simulink model "H_Bridge"  (R2022a)
settings: Solver=VariableStepAuto  StartTime=0.0  StopTime=.06  RelTol=1e-3
libraries: spsVoltageMeasurementLib x2, spsSeriesRLCBranchLib x1, slpidlib x1, spsPVArrayLib x1, spsCurrentMeasurementLib x1, spspowerguiLib x1
settings Model: Creator=micha  LastModifiedBy=micha
settings DataIOCC: ReturnWorkspaceOutputs=off

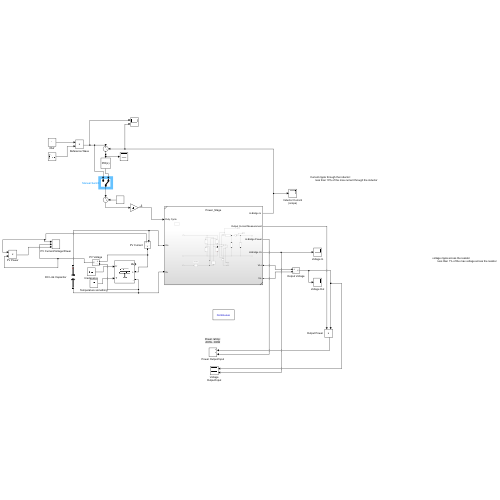
[thumbnail: Simulink's stored preview of the top-level diagram]
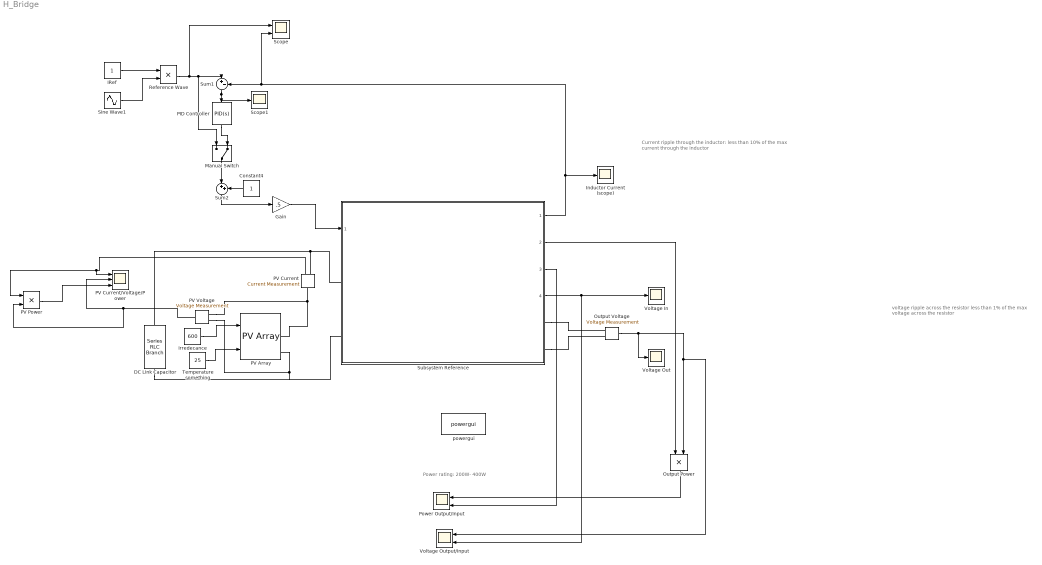
== system H_Bridge ==
  note: Current ripple through the inductor:
      | less than 10% of the max current through the inductor
  note: Power rating:
      | 200W- 400W
  note: voltage ripple across the resistor
      | less than 1% of the max voltage across the resistor
  Constant4 : Constant
  DC Link Capacitor : spsSeriesRLCBranchLib/Series RLC Branch  LConnTagsString=__new0  RConnTagsString=__new0  BranchType=C  Resistance=1  Inductance=1e-3  SetiL0=off  InitialCurrent=0  Capacitance=10000e-6  Setx0=off  InitialVoltage=0  Measurements=None
  Gain : Gain  Gain=.5
  IRef : Constant
  Inductor Current (scope) : Scope
  Irredecance : Constant  Value=600
  Manual Switch : ManualSwitch  CurrentSetting=0
  Output Power : Product
  Output Voltage : spsVoltageMeasurementLib/Voltage Measurement  PhasorSimulation=off  OutputType=Complex  PSBequivalent=0
  PID Controller : slpidlib/PID Controller  Controller=PID  Form=Parallel  TimeDomain=Continuous-time  UseExternalTs=off  SampleTime=-1  IntegratorMethod=Forward Euler  FilterMethod=Forward Euler  ControllerParametersSource=internal  P=1.59324162763222  I=2728.30196646129  UseKiTs=off  D=-8.00314894182289e-05  N=3055.81955398126  UseFilter=on  TunerSelectOption=Transfer Function Based (PID Tuner App)  InitialConditionSource=internal  InitialConditionForIntegrator=0  InitialConditionForFilter=0  DifferentiatorICPrevScaledInput=0  ExternalReset=none  TrackingMode=off  Kt=1  LimitOutput=off  SatLimitsSource=internal  UpperSaturationLimit=inf  LowerSaturationLimit=-inf  LinearizeAsGain=on  AntiWindupMode=none  Kb=1  POutMin=[]  POutMax=[]  IOutMin=[]  IOutMax=[]  DOutMin=[]  DOutMax=[]  NOutMin=[]  NOutMax=[]  SumOutMin=[]  SumOutMax=[]  SaturationOutMin=[]  SaturationOutMax=[]  PParamMin=[]  PParamMax=[]  IParamMin=[]  IParamMax=[]  DParamMin=[]  DParamMax=[]  NParamMin=[]  NParamMax=[]  KbParamMin=[]  KbParamMax=[]  KtParamMin=[]  KtParamMax=[]  KbOutMin=[]  KbOutMax=[]  KtOutMin=[]  KtOutMax=[]  IntegratorOutMin=[]  IntegratorOutMax=[]  FilterOutMin=[]  FilterOutMax=[]  SumI1OutMin=[]  SumI1OutMax=[]  SumI2OutMin=[]  SumI2OutMax=[]  SumI3OutMin=[]  SumI3OutMax=[]  SumI4OutMin=[]  SumI4OutMax=[]  SumDOutMin=[]  SumDOutMax=[]  DifferentiatorOutMin=[]  DifferentiatorOutMax=[]  FilterDiffOutCoefMin=[]  FilterDiffOutCoefMax=[]  ReciprocalOutMin=[]  ReciprocalOutMax=[]  SumDenOutMin=[]  SumDenOutMax=[]  SumNumOutMin=[]  SumNumOutMax=[]  DivideOutMin=[]  DivideOutMax=[]  UdiffTsProdOutMin=[]  UdiffTsProdOutMax=[]  NTsProdOutMin=[]  NTsProdOutMax=[]  UintegralTsProdOutMin=[]  UintegralTsProdOutMax=[]  UngainTsProdOutMin=[]  UngainTsProdOutMax=[]  IntegratorContinuousStateAttributes=''  IntegratorStateMustResolveToSignalObject=off  IntegratorRTWStateStorageClass=Auto  FilterContinuousStateAttributes=''  FilterStateMustResolveToSignalObject=off  FilterRTWStateStorageClass=Auto  ParallelPVariant=InternalParameters  IdealPVariant=Disabled  IVariant=InternalParameters  DVariant=InternalParameters  IntegratorVariant=Continuous  SatVariant=Disabled  AWVariant=Passthrough  PCopyVariant=Disabled  TRVariant=Disabled  FdbkBlocksVariant=Forward  IdealPFdbkVariant=Disabled  SatFdbkVariant=Disabled  DerivativeFilterVariant=ContFilter  NVariant=InternalParameters  NCopyVariant=Disabled  FilterICVariant=InternalICsFilter  IntegratorICVariant=InternalICs  ExternalResetVariant=Disabled  TRSumVariant=Passthrough  SumFdbkVariant=Disabled  SumVariant=Sum_PID  TsampFilterVariant=InternalTs  TsampNgainVariant=Passthrough  TsampIntegralVariant=Passthrough  ExternalSaturationOutDataTypeStr=Inherit: Same as second input  aMode=0
  PV Array : spsPVArrayLib/PV Array  Npar=1  Nser=1  PlotType=array @ 1000 W/m2 & specified temperatures  S_vec="[ 1000  500  100 ]"  Temp_C_vec="[ 45 25  ]"  ModuleName=SolarWorld Industries GmbH Sunmodule Plus SW 250 mono black  PlotWhenSelected=off  Pm=250.355  Ncell=60  Voc=37.8  Isc=8.28  Vm=31.1  Im=8.05  beta_Voc_pc=-0.313  alpha_Isc_pc=0.005  beta_Voc=-0.11831  alpha_Isc=0.000414  IL=8.3819  I0=4.5375e-11  nI=0.94533  Rsh=1469.9171  Rs=0.28491  RobustModel=off  RobustCellTemperature=313.3991  BAL=on  Tc=1e-6  Tfilter=5e-5
  PV Current : spsCurrentMeasurementLib/Current Measurement  PhasorSimulation=off  OutputType=Complex  PSBequivalent=0
  PV Current/Voltage/Power : Scope  NumInputPorts=3
  PV Power : Product
  PV Voltage : spsVoltageMeasurementLib/Voltage Measurement  PhasorSimulation=off  OutputType=Complex  PSBequivalent=0
  Power Output/Input : Scope  NumInputPorts=2
  Reference Wave : Product
  Scope : Scope  NumInputPorts=2
  Scope1 : Scope
  Sine Wave1 : Sin  Frequency=2*pi*60  SampleTime=0
  Subsystem Reference : Subsystem  ReferencedSubsystem=Power_Stage
  Sum1 : Sum  Inputs=|+-
  Sum2 : Sum  Inputs=|++
  Temperature something : Constant  Value=25
  Voltage Output/Input : Scope  NumInputPorts=2
  Voltage In : Scope
  Voltage Out : Scope
  powergui : spspowerguiLib/powergui  Priority=1  SimulationMode=Continuous  SampleTime=50e-6  frequency=60  Iterations=50  frequencyindice=0  Pbase=100e6  ErrMax=1e-4  UnitsV=kV  UnitsW=MW  buscounter=0  FunctionMessages=off  echomessages=off  EnableUseOfTLC=off  CurrentSourceSwitches=off  DisableSnubberDevices=off  DisableRonSwitches=off  DisableVfSwitches=off  DisplayEquations=off  AutomaticDiscreteSolvers=off  SolverType=Tustin/Backward Euler (TBE)  Interpol=off  ExternalGateDelay=off  methode=off  Ts=100  x0status=blocks  SPID=on  SwTol=0  HookPort=off  NonlinearTolerance=1e-4  nMaxIteration=100  ContinueOnMaxIteration=off  RestoreLinks=warning  ResistiveCurrentMeasurement=off  Frange=[0:2:500]  Ylog=off  Xlog=on  ShowGrid=off  save=off  variable=ZData  structure=0  ZoomFFT=off  StartTime=0.0  cycles=1  DisplayStyle=1  fundamental=60  FreqAxis=off  MaxFrequency=1000  frequencyindicesteady=1  RmsSteady=1  display=off
  wires:
  Output Voltage/1 -> Voltage Output/Input/1, Output Power/2, Voltage Out/1
  Output Power/1 -> Power Output/Input/1
  Subsystem Reference/3 -> Power Output/Input/2
  PV Current/1 -> PV Power/1, PV Current/Voltage/Power/1
  PV Voltage/1 -> PV Power/2, PV Current/Voltage/Power/2
  PV Power/1 -> PV Current/Voltage/Power/3
  Irredecance/1 -> PV Array/1
  Temperature something/1 -> PV Array/2
  Subsystem Reference/4 -> Voltage In/1, Voltage Output/Input/2
  Subsystem Reference/2 -> Output Power/1
  Reference Wave/1 -> Scope/1, Manual Switch/1, Sum1/1
  Gain/1 -> Subsystem Reference/1
  Sum2/1 -> Gain/1
  Manual Switch/1 -> Sum2/1
  PID Controller/1 -> Manual Switch/2
  Sine Wave1/1 -> Reference Wave/2
  Sum1/1 -> Scope1/1, PID Controller/1
  Subsystem Reference/1 -> Scope/2, Sum1/2, Inductor Current (scope)/1
  IRef/1 -> Reference Wave/1
  Constant4/1 -> Sum2/2
  connections:
  PV Array/RConn1 -- PV Voltage/LConn1 -- PV Current/LConn1
  PV Current/RConn1 -- Subsystem Reference/LConn1 -- DC Link Capacitor/LConn1
  PV Array/RConn2 -- DC Link Capacitor/RConn1 -- Subsystem Reference/LConn2 -- PV Voltage/LConn2
  Subsystem Reference/RConn1 -- Output Voltage/LConn1
  Subsystem Reference/RConn2 -- Output Voltage/LConn2
